simulink model "MagLev"  (R2024a)
settings: Solver=VariableStepAuto  StartTime=0.0  StopTime=10  RelTol=1e-3
values from neighbouring files (symbols this model uses):
  z0 = 0.01    [initial_conditions.m]    (also in initial_conditions_init.m = 0.015; parametersLoader.m)
settings Model: Creator=User  LastModifiedBy=Bocchio
settings DebuggingCC: UnconnectedInputMsg=warning  UnconnectedOutputMsg=warning  UnconnectedLineMsg=warning
settings ModelReferenceCC: EnableRefExpFcnMdlSchedulingChecks=on
settings RTWCC: GPUComputeCapability=3.5  DLArmComputeVersion=19.05

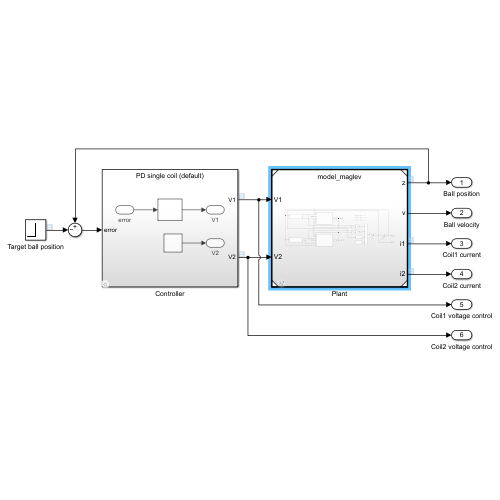
[thumbnail: Simulink's stored preview of the top-level diagram]
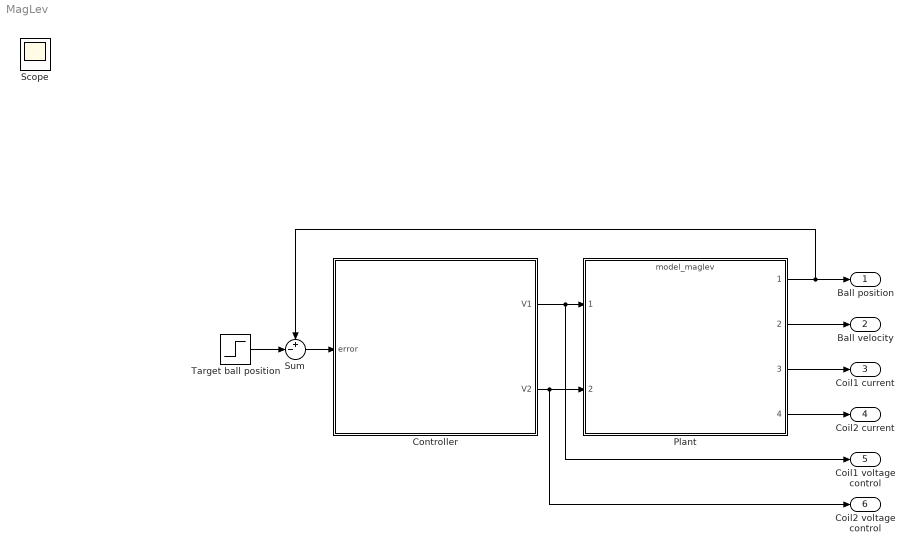
== system MagLev ==
  Controller : Subsystem  Variant=on
  Plant : ModelReference  ModelNameDialog=model_maglev.slx  SimulationMode=Normal  ModelReferenceVersion=1.52
  Sum : Sum  Inputs=+-|
  Target ball position : Step  Before=z0  After=z0 * (1+5/100)  SampleTime=0
  Ball position : Outport
  Ball velocity : Outport  Port=2
  Coil1 current : Outport  Port=3
  Coil2 current : Outport  Port=4
  Coil1 voltage control : Outport  Port=5
  Coil2 voltage control : Outport  Port=6
  Scope : Scope
  wires:
  Target ball position/1 -> Sum/2
  Controller/1(V1) -> Plant/1, Coil1 voltage control/1
  Sum/1 -> Controller/1(error)
  Plant/1 -> Sum/1, Ball position/1
  Controller/2(V2) -> Plant/2, Coil2 voltage control/1
  Plant/4 -> Coil2 current/1
  Plant/3 -> Coil1 current/1
  Plant/2 -> Ball velocity/1

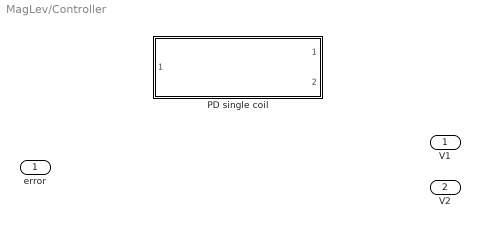
== system MagLev/Controller ==
  error : Inport
  PD single coil : Subsystem  VariantControl=(default)  ReferencedSubsystem=controller_PD_single_coil
  V1 : Outport
  V2 : Outport  Port=2
